simulink model "sample_system_MHE"  (R2022b)
settings: Solver=FixedStepDiscrete  StartTime=0.0  StopTime=T_final  FixedStep=T_sample  RelTol=1e-3
values from neighbouring files (symbols this model uses):
  A_bar_d = [0.9950 0.0998 ... (first row only)    [Run_model.m]    (also in prepare_trajectory_data.m)
  B_bar_d = [0.1 ... (first row only)    [Run_model.m]    (also in prepare_trajectory_data.m)
  C_obsv_d = [-0.48244804282  -0.463279461508; 0.0144227342104  -0.230554726046; 0.244765695792  -0.329721244669; 0.487562807757  0.730038636795; 0.684075320502  -0.191202440855; 0.0380669049625  0.232348391545]    [C_obsv_d.mat]    (also in sys_generation_WDS.m = C_obsv)
  D_obsv_d = zeros(n_meas,n_int)    [Run_model.m]    (also in prepare_trajectory_data.m; sys_generation_WDS.m = D_obsv)
  DE_MH = kron(eye(T),D_E)    [Run_model.m]
  E_MH = kron(eye(T),E)    [Run_model.m]
  H_pinv = pinv(H,0.001)    [Run_model.m]
  indicator = zeros(n_meas,1)    [Run_model.m]
  Lu = F-mpower(A_bar_d,T)*H0_pinv*H1    [Run_model.m]
  Ly = mpower(A_bar_d,T)*H0_pinv    [Run_model.m]
  n_alpha = size(HL_u,2)    [Run_model.m]
  n_meas = 6    [Run_model.m]    (also in prepare_trajectory_data.m; sys_generation_WDS.m = size(C_obsv,1); test.m = size(C,1))
  n_states = 10    [sys_generation_WDS.m]    (also in test.m = size(A,1))
  T = 5    [Run_model.m]    (also in prepare_trajectory_data.m)
  T_sample = 0.01    [Run_model.m]    (also in plot_error_table.m; prepare_trajectory_data.m; sys_generation_WDS.m; test.m)
  T_start_opt = load('Results/Data3.mat').T_start_opt    [plot_error_table.m]
  U0 = zeros(n_int,T+1)    [Run_model.m]
  x0 = [7;7]    [Run_model.m]    (also in prepare_trajectory_data.m; test.m = rand(n_states,1))
  Y0 = zeros(n_meas,T)    [Run_model.m]
undefined symbols (not defined in the file or in its folder): A_in1, A_in2, F, H0, H1
libraries: simulink x5
settings Model: Creator=Abelb  LastModifiedBy=Abelb
settings DebuggingCC: UnconnectedInputMsg=warning  UnconnectedOutputMsg=warning  UnconnectedLineMsg=warning
settings ModelReferenceCC: EnableRefExpFcnMdlSchedulingChecks=on
settings RTWCC: DLArmComputeVersion=19.05

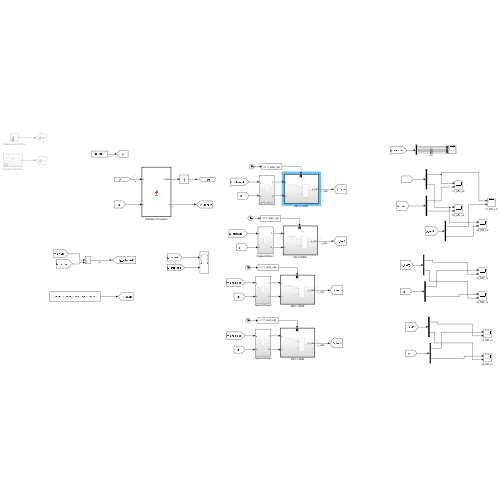
[thumbnail: Simulink's stored preview of the top-level diagram]
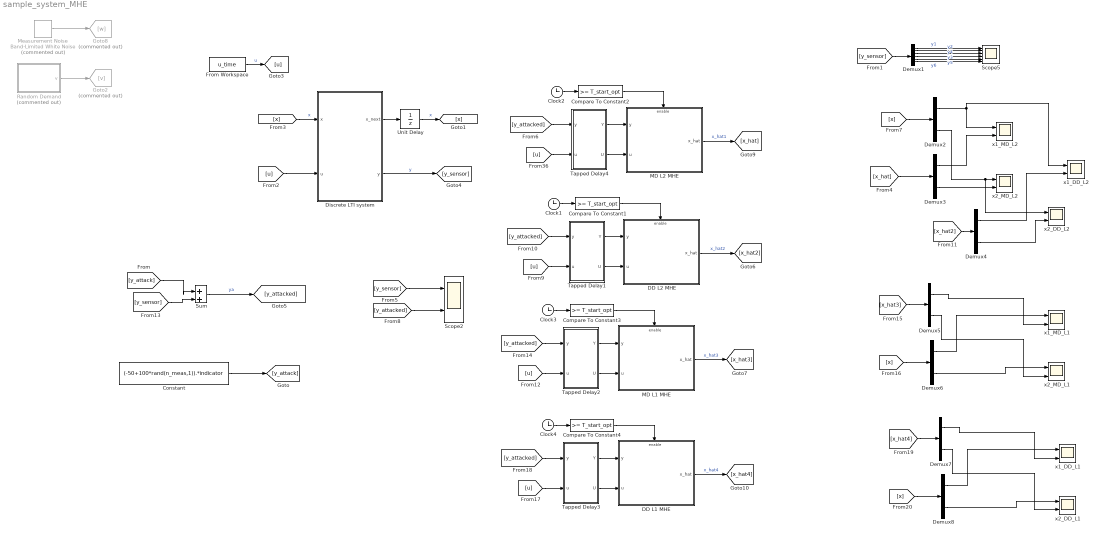
== system sample_system_MHE ==
  Clock{1..4} (4 alike) : Clock
  Compare To Constant{1..4} (4 alike) : simulink/Logic and Bit Operations/Compare To Constant  relop=>=  const=T_start_opt  OutDataTypeStr=boolean
  Constant : Constant  Value=(-50+100*rand(n_meas,1)).*indicator
  DD L1 MHE : Subsystem
  DD L2 MHE : Subsystem
  Demux1 : Demux  Outputs=6
  Demux{2..8} (7 alike) : Demux  Outputs=n_states
  Discrete LTI system : MATLAB Function  TreatAsAtomicUnit=on
  From Workspace : FromWorkspace  VariableName=u_time
  Goto2 : Goto  Commented=on  GotoTag=v
  Goto8 : Goto  Commented=on  GotoTag=w
  MD L1 MHE : Subsystem
  MD L2 MHE : Subsystem
  Measurement Noise : simulink/Sources/Band-Limited White Noise  Commented=on  Cov=[0.001]  Ts=T_sample  seed=[23341]
  Random Demand : Subsystem  Commented=on
  Scope2 : Scope  NumInputPorts=2
  Scope5 : Scope  NumInputPorts=6
  Sum : Sum  Inputs=|++
  Tapped Delay1 : Subsystem
  Tapped Delay2 : Subsystem
  Tapped Delay3 : Subsystem
  Tapped Delay4 : Subsystem
  Unit Delay : UnitDelay  InitialCondition=x0  SampleTime=-1  HasFrameUpgradeWarning=on
  x1_DD_L1 : Scope  NumInputPorts=2
  x1_DD_L2 : Scope  NumInputPorts=2
  x1_MD_L1 : Scope  NumInputPorts=2
  x1_MD_L2 : Scope  NumInputPorts=2
  x2_DD_L1 : Scope  NumInputPorts=2
  x2_DD_L2 : Scope  NumInputPorts=2
  x2_MD_L1 : Scope  NumInputPorts=2
  x2_MD_L2 : Scope  NumInputPorts=2
  wires:
  Discrete LTI system/1(x_next) -> Unit Delay/1
  Tapped Delay4/2(U) -> MD L2 MHE/2(u)
  MD L2 MHE/1(x_hat) -> [x_hat]  "x_hat1"
  [u] -> Tapped Delay4/2(u)
  Compare To Constant2/1 -> MD L2 MHE/Enable
  Tapped Delay4/1(Y) -> MD L2 MHE/1(y)
  Clock2/1 -> Compare To Constant2/1
  [x] -> Demux2/1
  Unit Delay/1 -> [x]  "x"
  [x] -> Discrete LTI system/1(x)  "x"
  [y_sensor] -> Scope2/1
  [y_attacked] -> Tapped Delay4/1(y)
  Constant/1 -> [y_attack]
  Measurement Noise/1 -> Goto8/1
  Random Demand/1(v) -> Goto2/1
  Discrete LTI system/2(y) -> [y_sensor]  "y"
  [y_sensor] -> Sum/2
  [y_attack] -> Sum/1
  Sum/1 -> [y_attacked]  "ya"
  [y_attacked] -> Scope2/2
  Demux1/2 -> Scope5/2  "y2"
  Demux1/5 -> Scope5/5  "y5"
  Demux1/3 -> Scope5/3  "y3"
  Demux1/1 -> Scope5/1  "y1"
  Demux1/6 -> Scope5/6  "y6"
  Demux1/4 -> Scope5/4  "y4"
  [y_sensor] -> Demux1/1
  From Workspace/1 -> [u]  "u"
  [u] -> Discrete LTI system/2(u)
  [x_hat] -> Demux3/1
  Demux2/1 -> x1_MD_L2/1, x1_DD_L2/1
  Demux3/1 -> x1_MD_L2/2
  Demux2/2 -> x2_DD_L2/1, x2_MD_L2/1
  Demux3/2 -> x2_MD_L2/2
  [y_attacked] -> Tapped Delay1/1(y)
  [u] -> Tapped Delay1/2(u)
  Compare To Constant1/1 -> DD L2 MHE/Enable
  Tapped Delay1/1(Y) -> DD L2 MHE/1(y)
  Clock1/1 -> Compare To Constant1/1
  DD L2 MHE/1(x_hat) -> [x_hat2]  "x_hat2"
  Tapped Delay1/2(U) -> DD L2 MHE/2(u)
  [x_hat2] -> Demux4/1
  Demux4/1 -> x1_DD_L2/2
  Demux4/2 -> x2_DD_L2/2
  [y_attacked] -> Tapped Delay2/1(y)
  [u] -> Tapped Delay2/2(u)
  Compare To Constant3/1 -> MD L1 MHE/Enable
  Tapped Delay2/1(Y) -> MD L1 MHE/1(y)
  Clock3/1 -> Compare To Constant3/1
  MD L1 MHE/1(x_hat) -> [x_hat3]  "x_hat3"
  Tapped Delay2/2(U) -> MD L1 MHE/2(u)
  [x_hat3] -> Demux5/1
  Demux5/1 -> x1_MD_L1/2
  Demux5/2 -> x2_MD_L1/2
  Demux6/2 -> x2_MD_L1/1
  [x] -> Demux6/1
  Demux6/1 -> x1_MD_L1/1
  [y_attacked] -> Tapped Delay3/1(y)
  [u] -> Tapped Delay3/2(u)
  Compare To Constant4/1 -> DD L1 MHE/Enable
  Tapped Delay3/1(Y) -> DD L1 MHE/1(y)
  Clock4/1 -> Compare To Constant4/1
  DD L1 MHE/1(x_hat) -> [x_hat4]  "x_hat4"
  Tapped Delay3/2(U) -> DD L1 MHE/2(u)
  [x_hat4] -> Demux7/1
  [x] -> Demux8/1
  Demux8/1 -> x1_DD_L1/1
  Demux7/2 -> x2_DD_L1/2
  Demux8/2 -> x2_DD_L1/1
  Demux7/1 -> x1_DD_L1/2

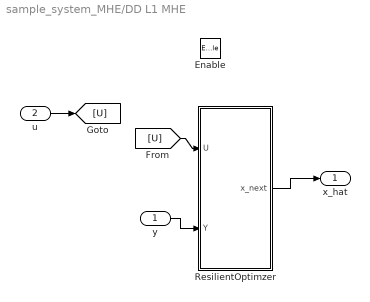
== system sample_system_MHE/DD L1 MHE ==
  y : Inport
  u : Inport  Port=2
  Enable : EnablePort
  ResilientOptimzer : MATLAB Function  TreatAsAtomicUnit=on
  x_hat : Outport
  wires:
  u/1 -> [U]
  y/1 -> ResilientOptimzer/2(Y)
  [U] -> ResilientOptimzer/1(U)
  ResilientOptimzer/1(x_next) -> x_hat/1

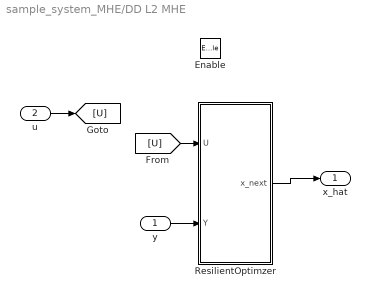
== system sample_system_MHE/DD L2 MHE ==
  y : Inport
  u : Inport  Port=2
  Enable : EnablePort
  ResilientOptimzer : MATLAB Function  TreatAsAtomicUnit=on
  x_hat : Outport
  wires:
  u/1 -> [U]
  y/1 -> ResilientOptimzer/2(Y)
  [U] -> ResilientOptimzer/1(U)
  ResilientOptimzer/1(x_next) -> x_hat/1

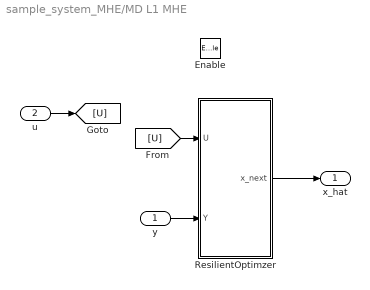
== system sample_system_MHE/MD L1 MHE ==
  y : Inport
  u : Inport  Port=2
  Enable : EnablePort
  ResilientOptimzer : MATLAB Function  TreatAsAtomicUnit=on
  x_hat : Outport
  wires:
  u/1 -> [U]
  y/1 -> ResilientOptimzer/2(Y)
  [U] -> ResilientOptimzer/1(U)
  ResilientOptimzer/1(x_next) -> x_hat/1

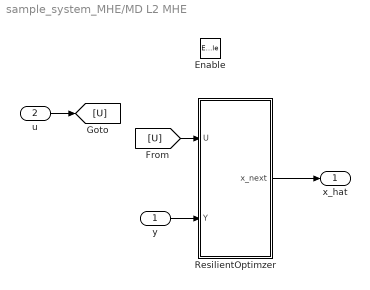
== system sample_system_MHE/MD L2 MHE ==
  y : Inport
  u : Inport  Port=2
  Enable : EnablePort
  ResilientOptimzer : MATLAB Function  TreatAsAtomicUnit=on
  x_hat : Outport
  wires:
  u/1 -> [U]
  y/1 -> ResilientOptimzer/2(Y)
  [U] -> ResilientOptimzer/1(U)
  ResilientOptimzer/1(x_next) -> x_hat/1

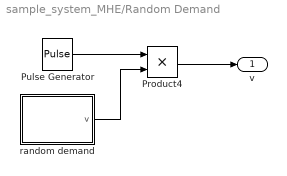
== system sample_system_MHE/Random Demand ==
  " random demand" : MATLAB Function  TreatAsAtomicUnit=on
  Product4 : Product
  Pulse Generator : DiscretePulseGenerator  Period=10  SampleTime=T_sample
  v : Outport
  wires:
  " random demand"/1(v) -> Product4/2
  Product4/1 -> v/1
  Pulse Generator/1 -> Product4/1

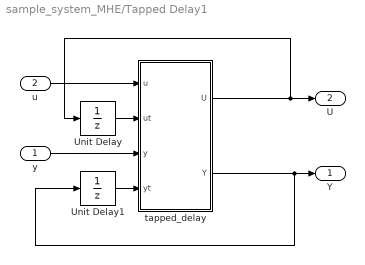
== system sample_system_MHE/Tapped Delay1 ==
  y : Inport
  u : Inport  Port=2
  Unit Delay : UnitDelay  InitialCondition=U0  SampleTime=-1  HasFrameUpgradeWarning=on
  Unit Delay1 : UnitDelay  InitialCondition=Y0  SampleTime=-1  HasFrameUpgradeWarning=on
  tapped_delay : MATLAB Function  TreatAsAtomicUnit=on
  Y : Outport
  U : Outport  Port=2
  wires:
  u/1 -> tapped_delay/1(u)
  y/1 -> tapped_delay/3(y)
  tapped_delay/1(U) -> Unit Delay/1, U/1
  tapped_delay/2(Y) -> Unit Delay1/1, Y/1
  Unit Delay/1 -> tapped_delay/2(ut)
  Unit Delay1/1 -> tapped_delay/4(yt)

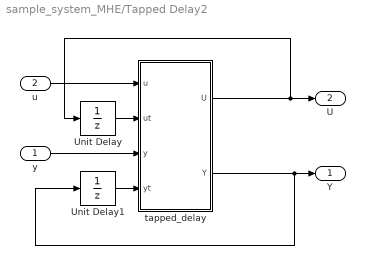
== system sample_system_MHE/Tapped Delay2 ==
  y : Inport
  u : Inport  Port=2
  Unit Delay : UnitDelay  InitialCondition=U0  SampleTime=-1  HasFrameUpgradeWarning=on
  Unit Delay1 : UnitDelay  InitialCondition=Y0  SampleTime=-1  HasFrameUpgradeWarning=on
  tapped_delay : MATLAB Function  TreatAsAtomicUnit=on
  Y : Outport
  U : Outport  Port=2
  wires:
  u/1 -> tapped_delay/1(u)
  y/1 -> tapped_delay/3(y)
  tapped_delay/1(U) -> Unit Delay/1, U/1
  tapped_delay/2(Y) -> Unit Delay1/1, Y/1
  Unit Delay/1 -> tapped_delay/2(ut)
  Unit Delay1/1 -> tapped_delay/4(yt)

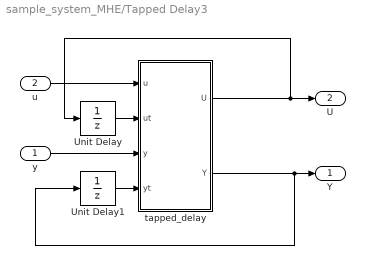
== system sample_system_MHE/Tapped Delay3 ==
  y : Inport
  u : Inport  Port=2
  Unit Delay : UnitDelay  InitialCondition=U0  SampleTime=-1  HasFrameUpgradeWarning=on
  Unit Delay1 : UnitDelay  InitialCondition=Y0  SampleTime=-1  HasFrameUpgradeWarning=on
  tapped_delay : MATLAB Function  TreatAsAtomicUnit=on
  Y : Outport
  U : Outport  Port=2
  wires:
  u/1 -> tapped_delay/1(u)
  y/1 -> tapped_delay/3(y)
  tapped_delay/1(U) -> Unit Delay/1, U/1
  tapped_delay/2(Y) -> Unit Delay1/1, Y/1
  Unit Delay/1 -> tapped_delay/2(ut)
  Unit Delay1/1 -> tapped_delay/4(yt)

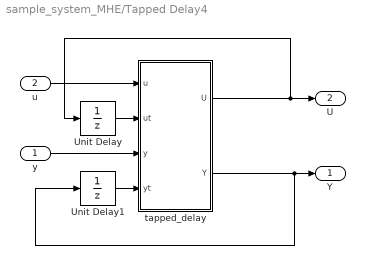
== system sample_system_MHE/Tapped Delay4 ==
  y : Inport
  u : Inport  Port=2
  Unit Delay : UnitDelay  InitialCondition=U0  SampleTime=-1  HasFrameUpgradeWarning=on
  Unit Delay1 : UnitDelay  InitialCondition=Y0  SampleTime=-1  HasFrameUpgradeWarning=on
  tapped_delay : MATLAB Function  TreatAsAtomicUnit=on
  Y : Outport
  U : Outport  Port=2
  wires:
  u/1 -> tapped_delay/1(u)
  y/1 -> tapped_delay/3(y)
  tapped_delay/1(U) -> Unit Delay/1, U/1
  tapped_delay/2(Y) -> Unit Delay1/1, Y/1
  Unit Delay/1 -> tapped_delay/2(ut)
  Unit Delay1/1 -> tapped_delay/4(yt)

== matlab function sample_system_MHE/DD L1 MHE/ResilientOptimzer ==
  data: x_next output; U input; Y input; A_in1 parameter; A_in2 parameter; n_states parameter; E_MH parameter; T parameter; n_alpha parameter; DE_MH parameter
function x_next   = fcn(U,Y, A_in1,A_in2, n_states,E_MH, T, n_alpha, DE_MH)    % DD L1
%% DD L1
%% function [x_next,r]  = fcn(U,Y, Aeq,n_states,E_MH,T, DE_MH, n_alpha, CE_MH)
% vectorized
u_local = U(2:end);
u = u_local(:);
y = Y(:);

x_next = zeros(n_states,1);

coder.extrinsic('DD_L1_MHE');
x_next(:) = DD_L1_MHE(y,u,T,A_in1, A_in2,n_states,E_MH,DE_MH,n_alpha);

== matlab function sample_system_MHE/Random Demand/ random demand ==
  data: v output; n_states parameter
function v = fcn(n_states)

v = 0.3*rand(n_states,1);

== matlab function sample_system_MHE/Tapped Delay3/tapped_delay ==
  data: u input; U output; ut input; y input; yt input; Y output
function [U,Y] = fcn(u,ut,y,yt)
%% tapped_delay_array
% shift columns from tapped matrix to the left and appends most recent
% vector to the last column
%%% input
ut(1:end-1) = ut(2:end);
ut(end) = u;
U = ut;
%%% output
yt(:,1:end-1) = yt(:,2:end);
yt(:,end) = y;
Y = yt;

== matlab function sample_system_MHE/Discrete LTI system ==
  data: x input; x_next output; u input; y output; A_bar_d parameter; C_obsv_d parameter; B_bar_d parameter; D_obsv_d parameter
function [x_next,y] = fcn(x,u,A_bar_d,C_obsv_d,B_bar_d,D_obsv_d)
% Discrete state-space model for system

x_next = A_bar_d*x + B_bar_d*u;

y = C_obsv_d*x + D_obsv_d*u;

== matlab function sample_system_MHE/Tapped Delay4/tapped_delay ==
  data: u input; U output; ut input; y input; yt input; Y output
function [U,Y] = fcn(u,ut,y,yt)
%% tapped_delay_array
% shift columns from tapped matrix to the left and appends most recent
% vector to the last column
%%% input
ut(1:end-1) = ut(2:end);
ut(end) = u;
U = ut;
%%% output
yt(:,1:end-1) = yt(:,2:end);
yt(:,end) = y;
Y = yt;

== matlab function sample_system_MHE/MD L2 MHE/ResilientOptimzer ==
  data: x_next output; U input; Y input; Ly parameter; Lu parameter; n_states parameter
function x_next    = fcn(U,Y, Ly, Lu,n_states)                                 % MD L2  
% function [x_next,r]  = fcn(U,Y,T, H0,H1,F,A_bar_d,n_states)                            % MD L1
% function [x_next,r]  = fcn(U,Y, Aeq,n_states,E_MH,T, CE_MH, n_alpha, DE_MH)          % DD L2, DD L1
% function [x_next,r]  = fcn(U,Y, A_in1,A_in2, n_states,E_MH,T, CE_MH, n_alpha, DE_MH)    % DD L1

%% MD L2
%% function [x_next,r]  = fcn(U,Y, Ly, Lu,H0_perp, H1)   
% vectorized
u_local = U(1:end-1);
u = u_local(:);
y = Y(:);

x_next = zeros(n_states,1);
x_next(:) = Ly*y +Lu*u ;


%% DD L2
%% function [x_next,r]  = fcn(U,Y, Aeq,n_states,E_MH,T, DE_MH, n_alpha, CE_MH)
% % vectorized
% u_local = U(:,2:end);
% u = u_local(:);
% y = Y(:);
% 
% x_next = zeros(n_states,1);
% r = zeros(size(y,1),1);
% 
% coder.extrinsic('DD_L2_MHE');
% [x_next(:)] = DD_L2_MHE(y,u,T,Aeq,n_states,E_MH,CE_MH,DE_MH,n_alpha);


%% MD L1
%% function [x_next,r]  = fcn(U,Y,T, H0,H1,F,A_bar_d,n_states) 
% % vectorized
% u_local = U(:,1:end-1);
% u = u_local(:);
% y = Y(:);
% 
% x_next = zeros(n_states,1);
% r = zeros(size(y,1),1);
% 
% coder.extrinsic('L1_MHE');
% [x_next(:),r(:)] = L1_MHE(y,u,T,H0,H1,F,A_bar_d,n_states);


%% DD L1
%% function [x_next,r]  = fcn(U,Y, Aeq,n_states,E_MH,T, DE_MH, n_alpha, CE_MH)
% % vectorized
% u_local = U(:,2:end);
% u = u_local(:);
% y = Y(:);
% 
% x_next = zeros(n_states,1);
% r = zeros(size(y,1),1);
% 
% coder.extrinsic('DD_L1_MHE');
% [x_next(:)] = DD_L1_MHE(y,u,T,A_in1, A_in2,n_states,E_MH,CE_MH,DE_MH,n_alpha);

== matlab function sample_system_MHE/DD L2 MHE/ResilientOptimzer ==
  data: x_next output; U input; Y input; H_pinv parameter; n_states parameter; E_MH parameter; T parameter; DE_MH parameter
function x_next   = fcn(U,Y, H_pinv,n_states,E_MH,T,DE_MH)          
%% DD L2
%% function [x_next,r]  = fcn(U,Y, Aeq,n_states,E_MH,T, DE_MH, n_alpha, CE_MH)

% vectorized
u_local = U(1:end-1);
u = u_local(:);
y = Y(:);

x_next = zeros(n_states,1);

coder.extrinsic('DD_L2_MHE');
[x_next(:)] = DD_L2_MHE(y,u,T,H_pinv,n_states,E_MH,DE_MH);

== matlab function sample_system_MHE/Tapped Delay1/tapped_delay ==
  data: u input; U output; ut input; y input; yt input; Y output
function [U,Y] = fcn(u,ut,y,yt)
%% tapped_delay_array
% shift columns from tapped matrix to the left and appends most recent
% vector to the last column
%%% input
ut(1:end-1) = ut(2:end);
ut(end) = u;
U = ut;
%%% output
yt(:,1:end-1) = yt(:,2:end);
yt(:,end) = y;
Y = yt;

== matlab function sample_system_MHE/MD L1 MHE/ResilientOptimzer ==
  data: x_next output; U input; Y input; T parameter; H0 parameter; n_states parameter; H1 parameter; A_bar_d parameter; F parameter
function x_next   = fcn(U,Y,T, H0,n_states, H1, A_bar_d, F)                            % MD L1
%% MD L1
%% function [x_next]  = fcn(U,Y,T, H0,H1,F,A_bar_d,n_states) 
% vectorized
u_local = U(1:end-1);
u = u_local(:);
y = Y(:);

x_next = zeros(n_states,1);

coder.extrinsic('L1_MHE');
x_next(:) = L1_MHE(y,u,T,H0,H1,F,A_bar_d,n_states);

== matlab function sample_system_MHE/Tapped Delay2/tapped_delay ==
  data: u input; U output; ut input; y input; yt input; Y output
function [U,Y] = fcn(u,ut,y,yt)
%% tapped_delay_array
% shift columns from tapped matrix to the left and appends most recent
% vector to the last column
%%% input
ut(1:end-1) = ut(2:end);
ut(end) = u;
U = ut;
%%% output
yt(:,1:end-1) = yt(:,2:end);
yt(:,end) = y;
Y = yt;
